simulink model "main"  (Simulink 8.0)
settings: Solver=ode4  StartTime=0.0  StopTime=stop_time  FixedStep=step_time  RelTol=1e-3
values from neighbouring files (symbols this model uses):
  Exp_Lamda = 8.1    [main_1.m]
  mean_wind = 5    [main_1.m]
  R = 21.65    [main_1.m]
settings Model: Creator=dujiexian  LastModifiedBy=dujiexian
settings DebuggingCC: FcnCallInpInsideContextMsg=EnableAllAsWarning

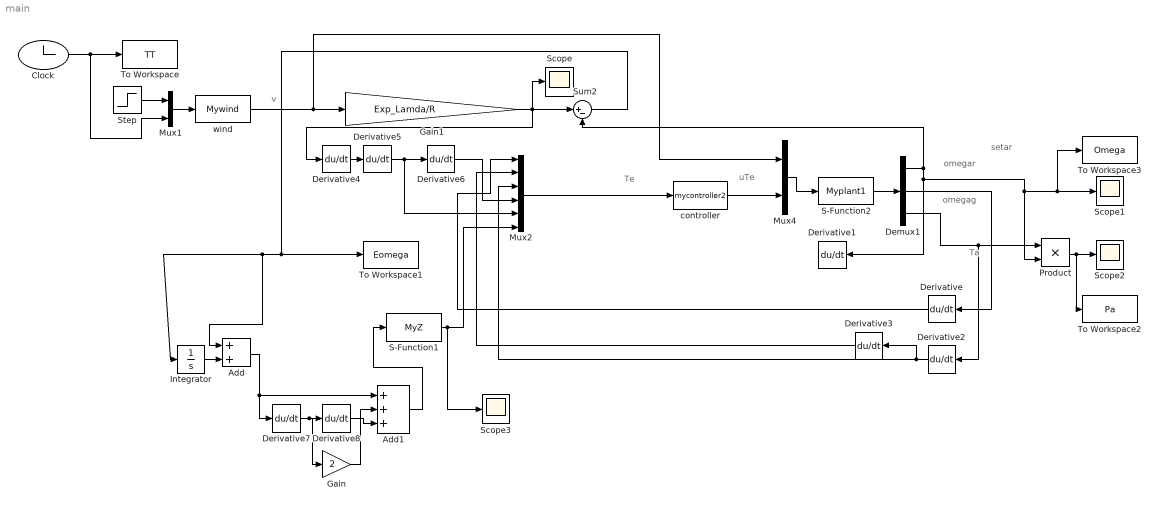
== system main ==
  note: Ta
  note: v
  note: Te
  note: uTe
  note: setar
  note: omegar
  note: omegag
  Add : Sum
  Add1 : Sum  Inputs=+++
  Clock : Clock
  Demux1 : Demux  Outputs=3
  Derivative{,1..8} (9 alike) : Derivative
  Gain : Gain  Gain=2
  Gain1 : Gain  Gain=Exp_Lamda/R
  Integrator : Integrator
  Mux1 : Mux  Inputs=2
  Mux2 : Mux  Inputs=6
  Mux4 : Mux  Inputs=2
  Product : Product  RndMeth=Zero
  S-Function1 : S-Function  FunctionName=MyZ  EnableBusSupport=off
  S-Function2 : S-Function  FunctionName=Myplant1  EnableBusSupport=off
  Scope{,1..3} (4 alike) : Scope
      Scope settings: YMin=4.1  YMax=5.7
      Scope1 settings: YMin=0  YMax=1.3
      Scope2 settings: YMin=0  YMax=1.3  SaveName=ScopeData2
      Scope3 settings: YMin=-100000  YMax=100000  SaveName=ScopeData3
  Step : Step  Time=0  After=mean_wind  SampleTime=0
  Sum2 : Sum  Inputs=|+-
  To Workspace : ToWorkspace  VariableName=TT  SampleTime=-1
  To Workspace1 : ToWorkspace  VariableName=Eomega  SampleTime=-1  SaveFormat=Timeseries
  To Workspace2 : ToWorkspace  VariableName=Pa  SampleTime=-1  SaveFormat=Timeseries
  To Workspace3 : ToWorkspace  VariableName=Omega  SampleTime=-1  SaveFormat=Timeseries
  "controller " : MATLABFcn  MATLABFcn=mycontroller2  OutputDimensions=1
  wind : MATLABFcn  MATLABFcn=Mywind
  wires:
  Clock/1 -> To Workspace/1, Mux1/2
  Step/1 -> Mux1/1
  Mux1/1 -> wind/1
  "controller "/1 -> Mux4/2
  S-Function2/1 -> Demux1/1
  Demux1/2 -> Derivative/1
  wind/1 -> Mux4/1, Gain1/1
  Gain1/1 -> Derivative4/1, Sum2/1, Scope/1
  Mux4/1 -> S-Function2/1
  Sum2/1 -> Add/1, Integrator/1, To Workspace1/1
  Demux1/1 -> To Workspace3/1, Scope1/1, Product/2, Derivative1/1, Sum2/2
  Demux1/3 -> Product/1, Derivative2/1
  Product/1 -> To Workspace2/1, Scope2/1
  Derivative2/1 -> Mux2/3, Derivative3/1
  Derivative4/1 -> Derivative5/1
  Derivative5/1 -> Derivative6/1, Mux2/5
  Derivative6/1 -> Mux2/4
  Mux2/1 -> "controller "/1
  Derivative/1 -> Mux2/1
  Derivative3/1 -> Mux2/2
  S-Function1/1 -> Scope3/1, Mux2/6
  Integrator/1 -> Add/2
  Add/1 -> Add1/1, Derivative7/1
  Derivative7/1 -> Gain/1, Derivative8/1
  Derivative8/1 -> Add1/3
  Add1/1 -> S-Function1/1
  Gain/1 -> Add1/2
